simulink model "Practica1_2"  (R2015a)
settings: Solver=ode45  StartTime=0.0  StopTime=8  RelTol=1e-3
settings Model: Creator=redes  LastModifiedBy=redes

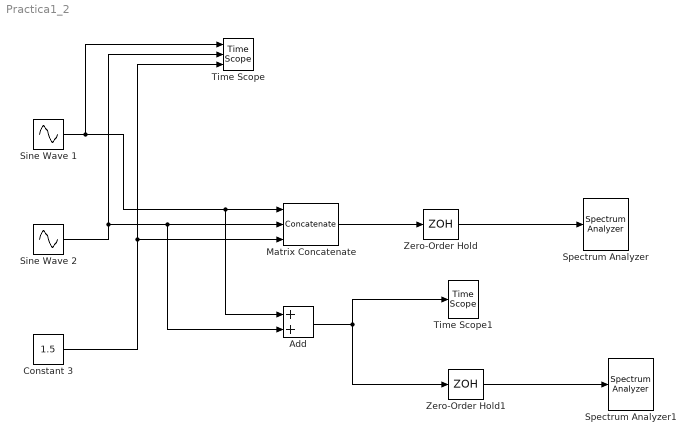
== system Practica1_2 ==
  Add : Sum
  Constant 3 : Constant  Value=1.5
  Matrix Concatenate : Concatenate  NumInputs=3  Mode=Multidimensional array  ConcatenateDimension=2
  Sine Wave 1 : Sin  Amplitude=1.5  Frequency=2*pi*30  SampleTime=0.0025
  Sine Wave 2 : Sin  Amplitude=3  Frequency=2*pi*10  SampleTime=0.0025
  Spectrum Analyzer : SpectrumAnalyzer
  Spectrum Analyzer1 : SpectrumAnalyzer
  Time Scope : TimeScope  DefaultConfigurationName=spbscopes.TimeScopeBlockCfg  NumInputPorts=3
  Time Scope1 : TimeScope  DefaultConfigurationName=spbscopes.TimeScopeBlockCfg
  Zero-Order Hold : ZeroOrderHold  SampleTime=0.0025
  Zero-Order Hold1 : ZeroOrderHold  SampleTime=0.0025
  wires:
  Sine Wave 1/1 -> Time Scope/1, Add/1, Matrix Concatenate/1
  Zero-Order Hold/1 -> Spectrum Analyzer/1
  Constant 3/1 -> Time Scope/3, Matrix Concatenate/3
  Sine Wave 2/1 -> Time Scope/2, Add/2, Matrix Concatenate/2
  Matrix Concatenate/1 -> Zero-Order Hold/1
  Zero-Order Hold1/1 -> Spectrum Analyzer1/1
  Add/1 -> Zero-Order Hold1/1, Time Scope1/1
